simulink model "FeedBackModel"  (R2015b)
settings: Solver=VariableStepAuto  StartTime=0.0  StopTime=20  RelTol=1e-3
libraries: cstblocks x2
settings Model: Creator=David  LastModifiedBy=David

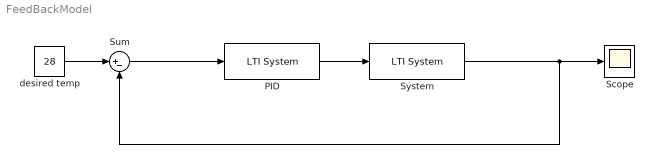
== system FeedBackModel ==
  PID : cstblocks/LTI System  sys=C  IC=[]
  Scope : Scope
  Sum : Sum  Inputs=|+-
  System : cstblocks/LTI System  sys=Plant2  IC=[]
  desired temp : Constant  Value=28
  wires:
  System/1 -> Scope/1, Sum/2
  desired temp/1 -> Sum/1
  PID/1 -> System/1
  Sum/1 -> PID/1
